simulink model "secondOrderActuator"  (R2020b)
settings: Solver=FixedStepAuto  StartTime=0.0  StopTime=10  FixedStep=0.01  RelTol=1e-3
model workspace (MAT data in the model file):
  Wn = 1.1
libraries: aerolibactuator x1
settings Model: Creator=Rafael.Casado  LastModifiedBy=usuario

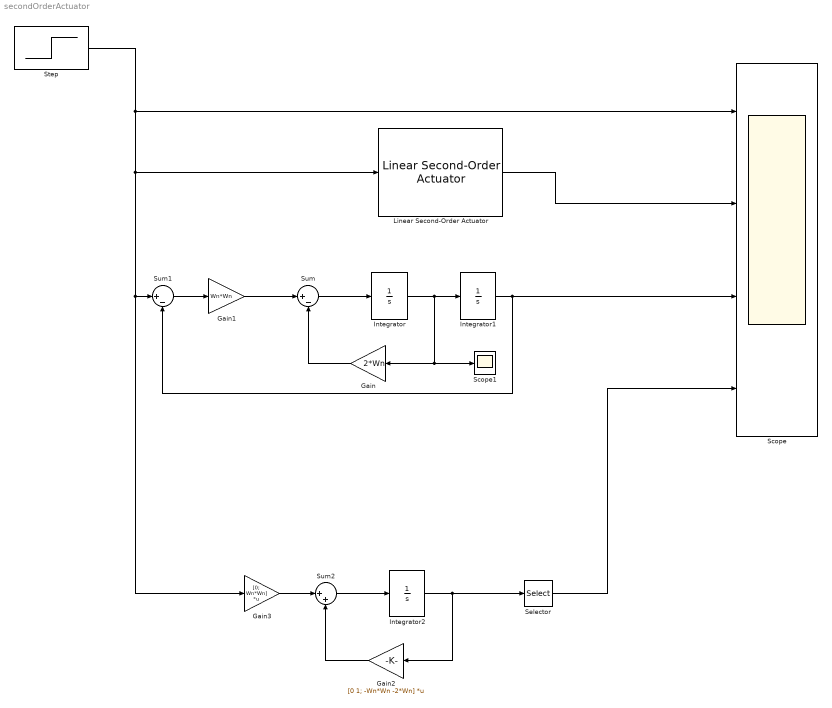
== system secondOrderActuator ==
  Gain : Gain  Gain=2*Wn
  Gain1 : Gain  Gain=Wn*Wn
  Gain2 : Gain  Gain=[0 1; -Wn*Wn -2*Wn]  Multiplication=Matrix(K*u)
  Gain3 : Gain  Gain=[0; Wn*Wn]  Multiplication=Matrix(K*u)
  Integrator : Integrator
  Integrator1 : Integrator  InitialCondition=82
  Integrator2 : Integrator  InitialCondition=[82; 0]
  Linear Second-Order Actuator : aerolibactuator/Linear Second-Order Actuator  wn_fin=Wn  z_fin=1  fin_act_0=82  fin_act_vel=0
      settings: SourceProductBaseCode=AE
  Scope : Scope  NumInputPorts=4
  Scope1 : Scope
  Selector : Selector  InputPortWidth=2  IndexOptions=Index vector (dialog)  Indices=[1]  OutputSizes=1
  Step : Step  Before=82  After=72  SampleTime=0
  Sum : Sum  Inputs=|+-
  Sum1 : Sum  Inputs=|+-
  Sum2 : Sum  Inputs=|++
  wires:
  Linear Second-Order Actuator/1 -> Scope/2
  Integrator/1 -> Integrator1/1, Scope1/1, Gain/1
  Sum/1 -> Integrator/1
  Gain/1 -> Sum/2
  Integrator1/1 -> Scope/3, Sum1/2
  Sum1/1 -> Gain1/1
  Gain1/1 -> Sum/1
  Step/1 -> Scope/1, Linear Second-Order Actuator/1, Gain3/1, Sum1/1
  Sum2/1 -> Integrator2/1
  Integrator2/1 -> Selector/1, Gain2/1
  Gain2/1 -> Sum2/2
  Gain3/1 -> Sum2/1
  Selector/1 -> Scope/4
